simulink model "psbdcdrive"  (Simulink 6.0)
settings: Solver=ode15s  SolverMode=SingleTasking  StartTime=0.0  StopTime=2.5
InitFcn:
  | powericon('psbinitsys',bdroot);
libraries: powerlib2 x12
settings Model: Creator=patrice  LastModifiedBy=batserve  ExtModeTrigMode=oneshot  ExtModeArmWhenConnect=off  ExtModeAutoUpdateStatusClock=off
settings DataIOCC: LimitDataPoints=off  SaveFinalState=on  SaveOutput=off  SaveTime=off  SignalLoggingName=sigsOut
settings OptimizationCC: BlockReduction=off  BooleanDataType=off
settings DebuggingCC: CheckExecutionContextPreStartOutputMsg=on  CheckExecutionContextRuntimeOutputMsg=on  SolverPrmCheckMsg=none  UnconnectedInputMsg=none  UnconnectedOutputMsg=none
settings HardwareCC: TargetUnknown=on
settings RTWCC: TemplateMakefile=grt_unix.tmf

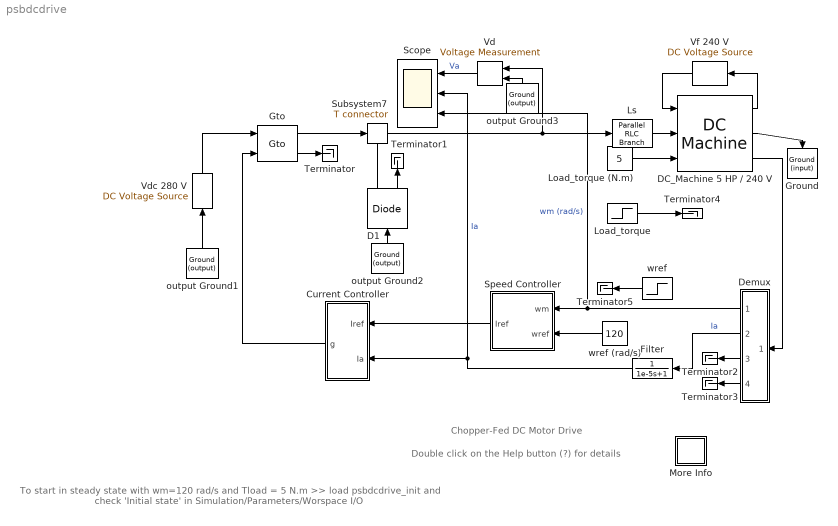
== system psbdcdrive ==
  note: Chopper-Fed DC Motor Drive
  note: To start in steady state with wm=120 rad/s and Tload = 5 N.m
      | >> load psbdcdrive_init
      | and check 'Initial state' in Simulation/Parameters/Worspace I/O
  note: Double click on the Help button (?) for details
  Current Controller : Subsystem  Orientation=left  mask{h=2}
      mask prompts: h "Hysteresis band (A)"
      mask help: Hysteresis Current Controller
      mask Display: plot(0,0,100,100,[45,45],[35,65],[55,55],[35,65],[45,65],[65,65],[35,55],[35,35])
  D1 : powerlib2/Power Electronics/Diode  Tag=PoWeRsYsTeMbLoCk  Orientation=up  Ron=0.05  Lon=5e-6  Vf=0.7  IC=0  Rs=Inf  Cs=0.1e-6  PSBOutputType=10
  DC_Machine 5 HP / 240 V : powerlib2/Machines/DC Machine  RLa="[0.5  0.01]"  RLf="[240  0]"  Laf=1.23  J=0.05  Bm=0.02  Tf=0  w0=1e-1  PSBOutputType=110
  Demux : Subsystem  Orientation=left
  Filter : TransferFcn  Orientation=left  Numerator=1  Denominator=[1e-5 1]
      mask Display: disp('Filter')
  Ground : powerlib2/Connectors/Ground (input)  Tag=PoWeRsYsTeMbLoCk  Orientation=down
  Gto : powerlib2/Power Electronics/Gto  Tag=PoWeRsYsTeMbLoCk  Ron=0.05  Lon=1e-6  Vf=1  Tf=1e-6  Tt=1e-6  IC=0  Rs=100  Cs=0.1e-6  PSBOutputType=10
  Load_torque (N.m) : Constant  Value=5
  "Load_torque " : Step  Time=1.2  Before=5  After=25  SampleTime=0
  Ls : powerlib2/Elements/Parallel RLC Branch  Tag=PoWeRsYsTeMbLoCk  a=inf  b=10e-03  c=0  mesure=None  PSBOutputType=1
  More Info : Subsystem
      mask Display: disp('?')
  Scope : Scope  NumInputPorts=3
      settings: TickLabels=on  YMin=-300~0~0  YMax=300~40~80  SaveName=var  Decimation=20
  Speed Controller : Subsystem  Orientation=left  mask(PI controller){Kp=1.6, Ki=16, Ilim=30}
      mask prompts: Kp "Proportional gain (Kp)"; Ki "Integral gain (Ki)"; Ilim "Current limit (A)"
      mask help: Proportional-Integral Speed Controller
      mask Display: plot(0,0,100,100,[35,35,65],[70,30,30],[35,65],[45,60])
  Subsystem7 : powerlib2/Connectors/T connector  Tag=PoWeRsYsTeMbLoCk  PSBOutputType=1
  Terminator{,1..5} (6 alike) : Terminator
      Terminator1 settings: Orientation=up
  Vd : powerlib2/Measurements/Voltage Measurement  Tag=PoWeRsYsTeMmEaSuReMeNt  Orientation=left  PhasorSimulation=off  OutputType=Magnitude  PSBOutputType=0  PSBequivalent=0
  "Vdc 280 V " : powerlib2/Electrical Sources/DC Voltage Source  Tag=PoWeRsYsTeMbLoCk  Orientation=up  V=280  mesure=None  PSBOutputType=1
  Vf 240 V : powerlib2/Electrical Sources/DC Voltage Source  Tag=PoWeRsYsTeMbLoCk  Orientation=left  V=240  mesure=None  PSBOutputType=1
  output Ground1 : powerlib2/Connectors/Ground (output)  Tag=PoWeRsYsTeMbLoCk  Orientation=up  PSBOutputType=1
  output Ground2 : powerlib2/Connectors/Ground (output)  Tag=PoWeRsYsTeMbLoCk  Orientation=up  PSBOutputType=1
  output Ground3 : powerlib2/Connectors/Ground (output)  Tag=PoWeRsYsTeMbLoCk  Orientation=up  PSBOutputType=1
  "wref " : Step  Orientation=left  Time=0.4  Before=120  After=160  SampleTime=0
  wref (rad/s) : Constant  Orientation=left  Value=120
  wires:
  D1/2 -> Terminator1/1
  Gto/2 -> Terminator/1
  output Ground2/1 -> D1/1
  D1/1 -> Subsystem7/Enable
  Gto/1 -> Subsystem7/1
  Current Controller/1(g) -> Gto/2
  "Vdc 280 V "/1 -> Gto/1
  output Ground1/1 -> "Vdc 280 V "/1
  Ls/1 -> DC_Machine 5 HP / 240 V/2
  Vf 240 V/1 -> DC_Machine 5 HP / 240 V/1
  Vd/1 -> Scope/1  "Va"
  Speed Controller/1(Iref) -> Current Controller/1(Iref)
  Subsystem7/1 -> Ls/1, Vd/1
  output Ground3/1 -> Vd/2
  Filter/1 -> Current Controller/2(Ia), Scope/2  "Ia"
  DC_Machine 5 HP / 240 V/2 -> Ground/1
  DC_Machine 5 HP / 240 V/1 -> Vf 240 V/1
  DC_Machine 5 HP / 240 V/3 -> Demux/1(m)
  Demux/1(wm) -> Speed Controller/1(wm), Scope/3  "wm (rad/s)"
  Demux/2(Ia) -> Filter/1  "Ia"
  Demux/4(Te) -> Terminator3/1
  Demux/3(If) -> Terminator2/1
  Load_torque (N.m)/1 -> DC_Machine 5 HP / 240 V/3
  wref (rad/s)/1 -> Speed Controller/2(wref)
  "Load_torque "/1 -> Terminator4/1
  "wref "/1 -> Terminator5/1

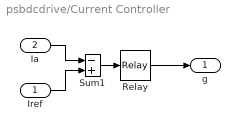
== system psbdcdrive/Current Controller ==
  Iref : Inport  Port=1  LatchInput=off
  Ia : Inport  Port=2  LatchInput=off
  Relay : Relay  OnSwitchValue=h/2  OffSwitchValue=-h/2
  Sum1 : Sum  Inputs=-+  SaturateOnIntegerOverflow=on  InputSameDT=on
  g : Outport  InitialOutput=0
  wires:
  Sum1/1 -> Relay/1
  Relay/1 -> g/1
  Ia/1 -> Sum1/1
  Iref/1 -> Sum1/2

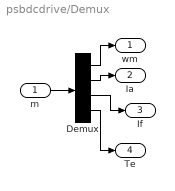
== system psbdcdrive/Demux ==
  m : Inport  Port=1  LatchInput=off
  Demux : Demux
  wm : Outport
  Ia : Outport  Port=2
  If : Outport  Port=3
  Te : Outport  Port=4
  wires:
  Demux/1 -> wm/1
  Demux/2 -> Ia/1
  m/1 -> Demux/1
  Demux/3 -> If/1
  Demux/4 -> Te/1

== system psbdcdrive/More Info ==
  note: Start the simulation. Observe the motor current, voltage, and speed during the starting on the scope.
      |
      | At the end of the simulation time (1.5 s), the system has attained its steady-state. The final state vector can
      | be saved by previously  selecting 'Workspace I/O/Save to workspace/Final state' in Simulation/Parameters window.
      | Once the simultion is finished save the xFinal variable into xInitial.
      |
      | Note : The initial conditions state vector xInitial to start with wm = 120 rad/s and Te = 5 N.m is stored in the psbdcdrive_init.mat file.
      |
      | Replace the constant wref and TL blocks by the two Simulink step functions with different starting times.
      | (Refence speed wref changed from 120 to 160 rad/s at t = 0.4 s and load torque changed from 5 to 25 N.m at  t= 2s)
      | Select  'Workspace I/O/Load from work space/Initial state' in Simulation parameters window to load the steady-state  vector xInitial.
      | Restart the simulation  and observe the drive response to successive changes in speed reference and load torque.
  note: Case study: Chopper-Fed DC Motor Drive
  note: Circuit Description
  note: Demonstration
  note: The DC motor is fed by the DC source through a chopper which consists of GTO thyristor Th1
      | and free-wheeling diode D1. The motor drives a mechanical load characterized by inertia J, friction
      | coeficient B, and load torque TL.
      |
      | The hysteresis current controller compares the sensed current with the reference and generates
      | the trigger signal for the GTO thyristor to force the motor current to follow the reference.
      | The speed control loop uses a proportional-integral controller which produces the reference for the current loop.
      | Current and Voltage Measurement blocks provide signals for visualization purpose.
  note: H. Le-Huy (Universite Laval, Quebec)

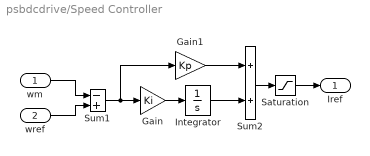
== system psbdcdrive/Speed Controller ==
  wm : Inport  Port=1  LatchInput=off
  wref : Inport  Port=2  LatchInput=off
  Gain : Gain  Gain=Ki  SaturateOnIntegerOverflow=on
  Gain1 : Gain  Gain=Kp  SaturateOnIntegerOverflow=on
  Integrator : Integrator  LimitOutput=on  UpperSaturationLimit=Ilim  LowerSaturationLimit=-Ilim
  Saturation : Saturate  UpperLimit=Ilim  LowerLimit=-Ilim
  Sum1 : Sum  Inputs=-+  SaturateOnIntegerOverflow=on  InputSameDT=on
  Sum2 : Sum  SaturateOnIntegerOverflow=on  InputSameDT=on
  Iref : Outport  InitialOutput=0
  wires:
  Saturation/1 -> Iref/1
  Sum2/1 -> Saturation/1
  Integrator/1 -> Sum2/2
  wref/1 -> Sum1/2
  wm/1 -> Sum1/1
  Sum1/1 -> Gain1/1, Gain/1
  Gain/1 -> Integrator/1
  Gain1/1 -> Sum2/1
